simulink model "controller"  (R2024b)
settings: Solver=VariableStepAuto  StartTime=0.0  StopTime=10.0  MaxStep=0.01  RelTol=1e-3
values from neighbouring files (symbols this model uses):
  CONTROL_PARAM = Simulink.Parameter(CONTROL_PARAM_VALUE)    [control_init.m]
undefined symbols (not defined in the file or in its folder): aL_sp, q, q_sp, timestamp, vforce, w
libraries: mqlib x3
settings Model: Creator=yangyu  LastModifiedBy=yangyu

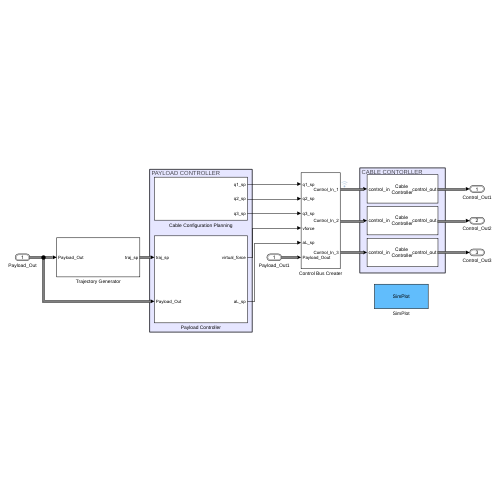
[thumbnail: Simulink's stored preview of the top-level diagram]
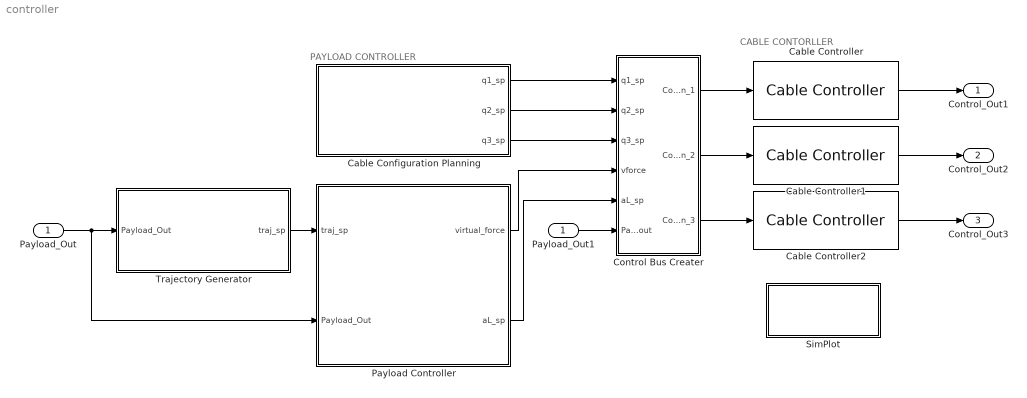
== system controller ==
  note: PAYLOAD CONTROLLER
  note: CABLE CONTORLLER
  Payload_Out1 : Inport  OutDataTypeStr=Bus: Payload_Out_Bus
  Cable Configuration Planning : Subsystem
  Cable Controller : mqlib/Cable Controller  Kq=CONTROL_PARAM.KQ  Kw=CONTROL_PARAM.KW  mi=CONTROL_PARAM.MASS_UAV  li=CONTROL_PARAM.CABLE_LEN
      link override Vertical Control/PID Controller: Controller=PI  TimeDomain=Discrete-time  ControllerParametersSource=internal  P=-Kq  I=-1
  Cable Controller1 : mqlib/Cable Controller  Kq=CONTROL_PARAM.KQ  Kw=CONTROL_PARAM.KW  mi=CONTROL_PARAM.MASS_UAV  li=CONTROL_PARAM.CABLE_LEN
  Cable Controller2 : mqlib/Cable Controller  Kq=CONTROL_PARAM.KQ  Kw=CONTROL_PARAM.KW  mi=CONTROL_PARAM.MASS_UAV  li=CONTROL_PARAM.CABLE_LEN
  Control Bus Creater : Subsystem
  Payload Controller : Subsystem
  Payload_Out : InportShadow  OutDataTypeStr=Bus: Payload_Out_Bus
  SimPlot : Subsystem
      settings: OpenFcn=run('simplot.m');
      mask Display: disp('SimPlot');
  Trajectory Generator : Subsystem
  Control_Out1 : Outport  OutDataTypeStr=Bus: Control_Out_Bus
  Control_Out2 : Outport  Port=2  OutDataTypeStr=Bus: Control_Out_Bus
  Control_Out3 : Outport  Port=3  OutDataTypeStr=Bus: Control_Out_Bus
  wires:
  Trajectory Generator/1(traj_sp) -> Payload Controller/1(traj_sp)
  Payload_Out/1 -> Payload Controller/2(Payload_Out), Trajectory Generator/1(Payload_Out)
  Cable Configuration Planning/1(q1_sp) -> Control Bus Creater/1(q1_sp)
  Payload Controller/1(virtual_force) -> Control Bus Creater/4(vforce)
  Payload Controller/2(aL_sp) -> Control Bus Creater/5(aL_sp)
  Cable Configuration Planning/2(q2_sp) -> Control Bus Creater/2(q2_sp)
  Cable Configuration Planning/3(q3_sp) -> Control Bus Creater/3(q3_sp)
  Payload_Out1/1 -> Control Bus Creater/6(Payload_Oout)
  Control Bus Creater/1(Control_In_1) -> Cable Controller/1
  Control Bus Creater/2(Control_In_2) -> Cable Controller1/1
  Control Bus Creater/3(Control_In_3) -> Cable Controller2/1
  Cable Controller/1 -> Control_Out1/1
  Cable Controller1/1 -> Control_Out2/1
  Cable Controller2/1 -> Control_Out3/1

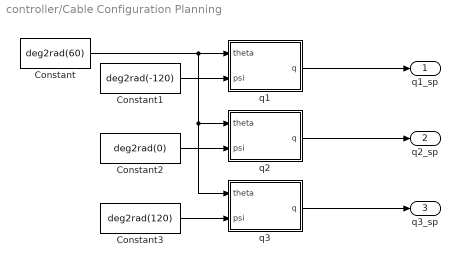
== system controller/Cable Configuration Planning ==
  Constant : Constant  Value=deg2rad(60)
  Constant1 : Constant  Value=deg2rad(-120)
  Constant2 : Constant  Value=deg2rad(0)
  Constant3 : Constant  Value=deg2rad(120)
  q1 : MATLAB Function  TreatAsAtomicUnit=on
  q2 : MATLAB Function  TreatAsAtomicUnit=on
  q3 : MATLAB Function  TreatAsAtomicUnit=on
  q1_sp : Outport
  q2_sp : Outport  Port=2
  q3_sp : Outport  Port=3
  wires:
  q2/1(q) -> q2_sp/1
  q3/1(q) -> q3_sp/1
  q1/1(q) -> q1_sp/1
  Constant/1 -> q1/1(theta), q2/1(theta), q3/1(theta)
  Constant1/1 -> q1/2(psi)
  Constant2/1 -> q2/2(psi)
  Constant3/1 -> q3/2(psi)

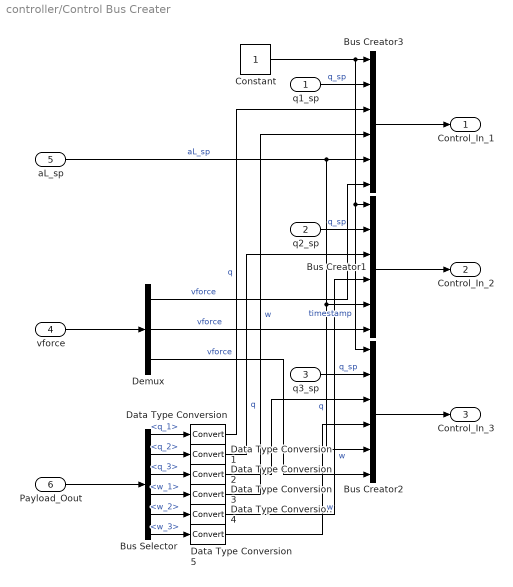
== system controller/Control Bus Creater ==
  q1_sp : Inport
  q2_sp : Inport  Port=2
  q3_sp : Inport  Port=3
  vforce : Inport  Port=4
  aL_sp : Inport  Port=5
  Payload_Oout : Inport  Port=6
  Bus Creator1 : BusCreator  Inputs=timestamp,q_sp,q,w,aL_sp,vforce  OutDataTypeStr=Bus: Control_In_Bus
  Bus Creator2 : BusCreator  Inputs=timestamp,q_sp,q,w,aL_sp,vforce  OutDataTypeStr=Bus: Control_In_Bus
  Bus Creator3 : BusCreator  Inputs=timestamp,q_sp,q,w,aL_sp,vforce  OutDataTypeStr=Bus: Control_In_Bus
  Bus Selector : BusSelector  OutputSignals=q_1,q_2,q_3,w_1,w_2,w_3
  Constant : Constant  OutDataTypeStr=uint32
  Data Type Conversion{,1..5} (6 alike) : DataTypeConversion  SaturateOnIntegerOverflow=off  RndMeth=Floor
  Demux : Demux  Outputs=3
  Control_In_1 : Outport
  Control_In_2 : Outport  Port=2
  Control_In_3 : Outport  Port=3
  wires:
  Demux/3 -> Bus Creator2/6  "vforce"
  Bus Selector/5 -> Data Type Conversion4/1  "<w_2>"
  vforce/1 -> Demux/1
  Bus Selector/6 -> Data Type Conversion5/1  "<w_3>"
  Bus Selector/3 -> Data Type Conversion2/1  "<q_3>"
  Payload_Oout/1 -> Bus Selector/1
  Demux/2 -> Bus Creator1/6  "vforce"
  Data Type Conversion1/1 -> Bus Creator1/3  "q"
  aL_sp/1 -> Bus Creator3/5, Bus Creator1/5, Bus Creator2/5  "aL_sp"
  Bus Creator1/1 -> Control_In_2/1
  Bus Creator2/1 -> Control_In_3/1
  q2_sp/1 -> Bus Creator1/2  "q_sp"
  q3_sp/1 -> Bus Creator2/2  "q_sp"
  Bus Creator3/1 -> Control_In_1/1
  q1_sp/1 -> Bus Creator3/2  "q_sp"
  Bus Selector/1 -> Data Type Conversion/1  "<q_1>"
  Data Type Conversion3/1 -> Bus Creator3/4  "w"
  Demux/1 -> Bus Creator3/6  "vforce"
  Constant/1 -> Bus Creator2/1, Bus Creator1/1, Bus Creator3/1  "timestamp"
  Data Type Conversion/1 -> Bus Creator3/3  "q"
  Bus Selector/2 -> Data Type Conversion1/1  "<q_2>"
  Data Type Conversion2/1 -> Bus Creator2/3  "q"
  Bus Selector/4 -> Data Type Conversion3/1  "<w_1>"
  Data Type Conversion4/1 -> Bus Creator1/4  "w"
  Data Type Conversion5/1 -> Bus Creator2/4  "w"

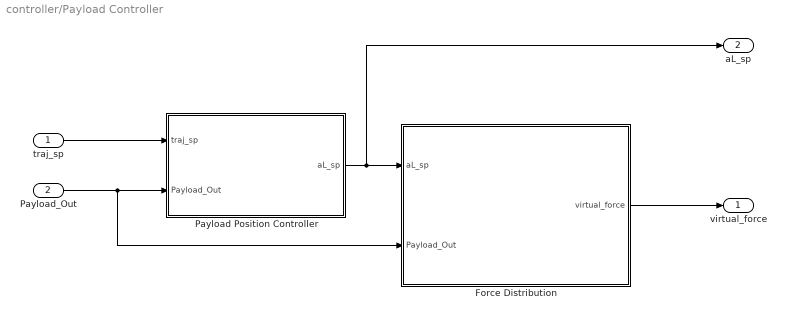
== system controller/Payload Controller ==
  traj_sp : Inport
  Payload_Out : Inport  Port=2
  Force Distribution : Subsystem
  Payload Position Controller : Subsystem
  virtual_force : Outport
  aL_sp : Outport  Port=2
  wires:
  Payload_Out/1 -> Force Distribution/2(Payload_Out), Payload Position Controller/2(Payload_Out)
  traj_sp/1 -> Payload Position Controller/1(traj_sp)
  Force Distribution/1(virtual_force) -> virtual_force/1
  Payload Position Controller/1(aL_sp) -> aL_sp/1, Force Distribution/1(aL_sp)

== system controller/SimPlot ==

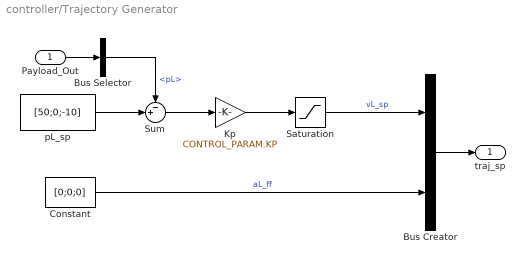
== system controller/Trajectory Generator ==
  Payload_Out : Inport
  Bus Creator : BusCreator  Inputs=2
  Bus Selector : BusSelector  OutputSignals=pL
  Constant : Constant  Value=[0;0;0]
  Kp : Gain  Gain=CONTROL_PARAM.KP
  Saturation : Saturate  UpperLimit=2  LowerLimit=-2
  Sum : Sum  Inputs=-+|
  pL_sp : Constant  Value=[50;0;-10]
  traj_sp : Outport
  wires:
  Saturation/1 -> Bus Creator/1  "vL_sp"
  Bus Creator/1 -> traj_sp/1
  pL_sp/1 -> Sum/2
  Payload_Out/1 -> Bus Selector/1
  Bus Selector/1 -> Sum/1  "<pL>"
  Sum/1 -> Kp/1
  Kp/1 -> Saturation/1
  Constant/1 -> Bus Creator/2  "aL_ff"

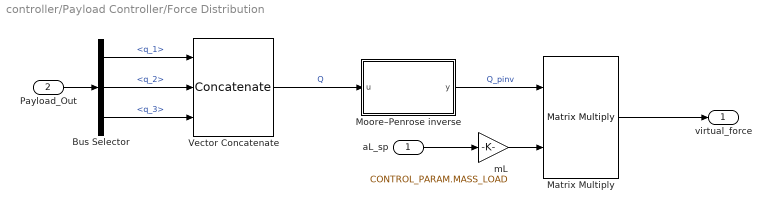
== system controller/Payload Controller/Force Distribution ==
  aL_sp : Inport
  Payload_Out : Inport  Port=2
  Bus Selector : BusSelector  OutputSignals=q_1,q_2,q_3
  Matrix Multiply : Product  Multiplication=Matrix(*)
  Moore–Penrose inverse : MATLAB Function  TreatAsAtomicUnit=on
  Vector Concatenate : Concatenate  NumInputs=3  Mode=Multidimensional array  ConcatenateDimension=2
  mL : Gain  Gain=CONTROL_PARAM.MASS_LOAD
  virtual_force : Outport
  wires:
  aL_sp/1 -> mL/1
  Bus Selector/1 -> Vector Concatenate/1  "<q_1>"
  Matrix Multiply/1 -> virtual_force/1
  Bus Selector/2 -> Vector Concatenate/2  "<q_2>"
  Vector Concatenate/1 -> Moore–Penrose inverse/1(u)  "Q"
  Payload_Out/1 -> Bus Selector/1
  Moore–Penrose inverse/1(y) -> Matrix Multiply/1  "Q_pinv"
  Bus Selector/3 -> Vector Concatenate/3  "<q_3>"
  mL/1 -> Matrix Multiply/2

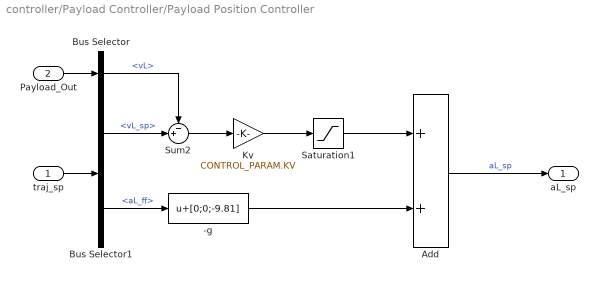
== system controller/Payload Controller/Payload Position Controller ==
  traj_sp : Inport
  Payload_Out : Inport  Port=2
  -g : Bias  Bias=[0;0;-9.81]  SaturateOnIntegerOverflow=off
  Add : Sum
  Bus Selector : BusSelector  OutputSignals=vL
  Bus Selector1 : BusSelector  OutputSignals=vL_sp,aL_ff
  Kv : Gain  Gain=CONTROL_PARAM.KV
  Saturation1 : Saturate  UpperLimit=1  LowerLimit=-1
  Sum2 : Sum  Inputs=-+|
  aL_sp : Outport
  wires:
  Sum2/1 -> Kv/1
  Bus Selector/1 -> Sum2/1  "<vL>"
  Bus Selector1/2 -> -g/1  "<aL_ff>"
  Bus Selector1/1 -> Sum2/2  "<vL_sp>"
  -g/1 -> Add/2
  Add/1 -> aL_sp/1  "aL_sp"
  Kv/1 -> Saturation1/1
  traj_sp/1 -> Bus Selector1/1
  Payload_Out/1 -> Bus Selector/1
  Saturation1/1 -> Add/1

== matlab function controller/Payload Controller/Force Distribution/Moore–Penrose inverse ==
  data: u input; y output
function y = fcn(u)

y = pinv(u);

== matlab function controller/Cable Configuration Planning/q2 ==
  data: theta input; q output; psi input
function q = fcn(theta, psi)

q = [-cos(psi) * cos(theta); -sin(psi) * cos(theta); sin(theta)];

== matlab function controller/Cable Configuration Planning/q3 ==
  data: theta input; q output; psi input
function q = fcn(theta, psi)

q = [-cos(psi) * cos(theta); -sin(psi) * cos(theta); sin(theta)];

== matlab function controller/Cable Configuration Planning/q1 ==
  data: theta input; q output; psi input
function q = fcn(theta, psi)

q = [-cos(psi) * cos(theta); -sin(psi) * cos(theta); sin(theta)];
